simulink model "pendulum_animation1"  (Simulink 8.2)
settings: Solver=ode45  StartTime=0.0  StopTime=10  RelTol=1e-3
undefined symbols (not defined in the file or in its folder): controller, drawPendulum, P
libraries: simulink x1
settings Model: Creator=beard  LastModifiedBy=aksha
settings OptimizationCC: InitFltsAndDblsToZero=on

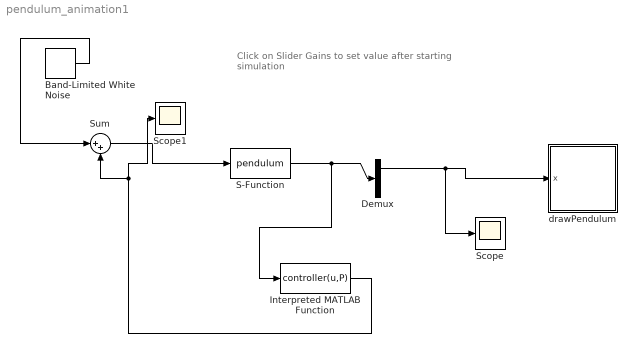
== system pendulum_animation1 ==
  note: Click on Slider Gains to set value
      | after starting simulation
  Band-Limited White Noise : simulink/Sources/Band-Limited White Noise  Cov=[0.1]  Ts=0.1  seed=[23341]
  Demux : Demux  Outputs=2
  Interpreted MATLAB Function : MATLABFcn  MATLABFcn=controller(u,P)
  S-Function : S-Function  FunctionName=pendulum  Parameters=P  EnableBusSupport=off
  Scope : Scope
  Scope1 : Scope
  Sum : Sum  Inputs=|++
  drawPendulum : Subsystem
      mask init:
      | % drawing parameters
      | L = 1;
      | gap = 0.01;
      | width = 1.0;
      | height = 0.1;
      mask Display: image(imread('tv.jpg'))
  wires:
  S-Function/1 -> Interpreted MATLAB Function/1, Demux/1
  Demux/1 -> Scope/1, drawPendulum/1(x)
  Interpreted MATLAB Function/1 -> Sum/2, Scope1/1
  Band-Limited White Noise/1 -> Sum/1
  Sum/1 -> S-Function/1

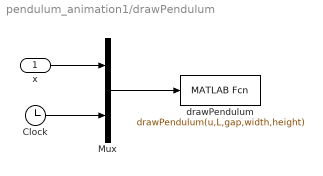
== system pendulum_animation1/drawPendulum ==
  x : Inport
  Clock : Clock
  Mux : Mux  Inputs=2
  drawPendulum : MATLABFcn  MATLABFcn=drawPendulum(u,L,gap,width,height)  OutputDimensions=0  SampleTime=0.1
  wires:
  Mux/1 -> drawPendulum/1
  x/1 -> Mux/1
  Clock/1 -> Mux/2
